simulink model "OBS6impedance"  (Simulink 7.4)
settings: Solver=ode45  StartTime=0.0  StopTime=8  MinStep=0.01  RelTol=1e-3
values from neighbouring files (symbols this model uses):
  Kact = eye(7)    [batchwamobs.m]
  Kd = Kp.^0.5*2    [WAMforcecontrol.m]    (also in batchwamobs.m = 50*eye(7); paralelcontrol2R.m = eye(n)*1000)
  Kp = 25*eye(7)    [batchwamobs.m]    (also in paralelcontrol2R.m = eye(n)*2500)
undefined symbols (not defined in the file or in its folder): Kf, Kif, Mdi, model1, model2, model3, model4, model5, model6, ncalculest, p560, uextgeneratorwall
libraries: roblocks x2
settings Model: Creator=acolome  LastModifiedBy=acolome

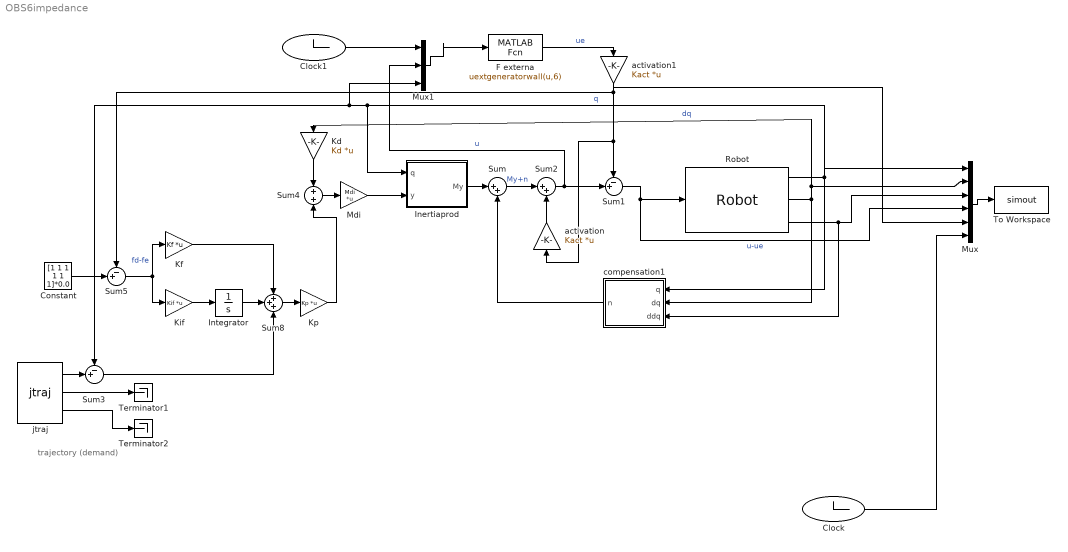
== system OBS6impedance ==
  note: trajectory
      | (demand)
  Clock : Clock
      settings: Decimation=100
  Clock1 : Clock
      settings: Decimation=100
  Constant : Constant  Value=[1 1 1 1 1 1]*0.0  OutDataType=fixdt(1, 16)  OutScaling=2^0
  F externa : MATLABFcn  MATLABFcn=uextgeneratorwall(u,6)  OutputDimensions=6
  Inertiaprod : Subsystem  mask{robot=p560, g=[0 0 9.81]}
      mask prompts: robot "Robot Object"; g "Gravity"
      mask init:
      | n=robot.n
      mask Display:
      | port_label('output',1,'M(q)y')
      | 
      | port_label('input', 1, 'q')
      | port_label('input', 2, 'y')
  Integrator : Integrator
  Kd : Gain  Gain=Kd  Multiplication=Matrix(K*u)  SaturateOnIntegerOverflow=on  OutDataTypeStr=Inherit: Same as input  ParamDataTypeStr=Inherit: Same as input
  Kf : Gain  Gain=Kf  Multiplication=Matrix(K*u)  SaturateOnIntegerOverflow=on  OutDataTypeStr=Inherit: Same as input  ParamDataTypeStr=Inherit: Same as input
  Kif : Gain  Gain=Kif  Multiplication=Matrix(K*u)  SaturateOnIntegerOverflow=on  OutDataTypeStr=Inherit: Same as input  ParamDataTypeStr=Inherit: Same as input
  Kp : Gain  Gain=Kp  Multiplication=Matrix(K*u)  SaturateOnIntegerOverflow=on  OutDataTypeStr=Inherit: Same as input  ParamDataTypeStr=Inherit: Same as input
  Mdi : Gain  Gain=Mdi  Multiplication=Matrix(K*u)  SaturateOnIntegerOverflow=on  OutDataTypeStr=Inherit: Same as input  ParamDataTypeStr=Inherit: Same as input
  Mux : Mux  Inputs=6
  Mux1 : Mux  Inputs=3
  Robot : roblocks/Robot  SystemSampleTime=-1  robot=p560  q0=[0 0 0 0 0 pi/20]*0
  Sum : Sum  Inputs=|++  OutDataType=fixdt(1, 16)  OutScaling=2^0
  Sum1 : Sum  Inputs=-+|  OutDataType=fixdt(1, 16)  OutScaling=2^0
  Sum2 : Sum  Inputs=|++  OutDataType=fixdt(1, 16)  OutScaling=2^0
  Sum3 : Sum  Inputs=-+|  SaturateOnIntegerOverflow=on  InputSameDT=on  OutDataTypeStr=Inherit: Same as first input
  Sum4 : Sum  SaturateOnIntegerOverflow=on  InputSameDT=on  OutDataTypeStr=Inherit: Same as first input
  Sum5 : Sum  Inputs=-+|  SaturateOnIntegerOverflow=on  InputSameDT=on  OutDataTypeStr=Inherit: Same as first input
  Sum8 : Sum  Inputs=+++  SaturateOnIntegerOverflow=on  InputSameDT=on  OutDataTypeStr=Inherit: Same as first input
  Terminator1 : Terminator
  Terminator2 : Terminator
  To Workspace : ToWorkspace  VariableName=simout  SampleTime=-1  SaveFormat=Array
  activation : Gain  Gain=Kact  Multiplication=Matrix(K*u)  SaturateOnIntegerOverflow=on  OutDataTypeStr=Inherit: Same as input  ParamDataTypeStr=Inherit: Same as input
  activation1 : Gain  Gain=Kact  Multiplication=Matrix(K*u)  SaturateOnIntegerOverflow=on  OutDataTypeStr=Inherit: Same as input  ParamDataTypeStr=Inherit: Same as input
  compensation1 : Subsystem  mask{robot=p560, g=[0 0 9.81], model1=model1, model2=model2, model3=model3, model4=model4, model5=model5, model6=model6}
      mask prompts: robot "Robot Object"; g "Gravity"; model1 "n1"; model2 "n2"; model3 "n3"; model4 "n4"; model5 "n5"; model6 "n6"
      mask init:
      | n=robot.n
      mask Display:
      | port_label('output',1,'n(q,dq)')
      | 
      | port_label('input', 1, 'q')
      | port_label('input', 2, 'dq')
      | port_label('input', 3, 'ddq')
  jtraj : roblocks/jtraj  SystemSampleTime=-1  q0=[0 0 0 0 0 pi/20]*0  qf=[1 1 1 1 1 1]  tmax=3
      link override MATLAB Fcn: MATLABFcn=squeeze(interp1(t,q,u))
      link override MATLAB Fcn1: MATLABFcn=squeeze(interp1(t,qd,u))
      link override MATLAB Fcn2: MATLABFcn=squeeze(interp1(t,qdd,u))
  wires:
  Mux/1 -> To Workspace/1
  jtraj/1 -> Sum3/2
  Robot/1 -> Mux/1, compensation1/1(q), Inertiaprod/1(q), Sum3/1, Mux1/3  "q"
  Robot/2 -> compensation1/2(dq), Mux/2, Kd/1  "dq"
  Robot/3 -> Mux/3, compensation1/3(ddq)
  compensation1/1(n) -> Sum/2
  Sum1/1 -> Robot/1, Mux/4  "u-ue"
  Inertiaprod/1(My) -> Sum/1
  Sum/1 -> Sum2/1  "My+n"
  Sum2/1 -> Sum1/2, Mux1/2  "u"
  F externa/1 -> activation1/1  "ue"
  activation1/1 -> Sum5/1, Sum1/1, activation/1, Mux/5
  activation/1 -> Sum2/2
  Constant/1 -> Sum5/2
  Sum5/1 -> Kf/1, Kif/1  "fd-fe"
  Kif/1 -> Integrator/1
  Kf/1 -> Sum8/1
  Integrator/1 -> Sum8/2
  jtraj/2 -> Terminator1/1
  jtraj/3 -> Terminator2/1
  Sum3/1 -> Sum8/3
  Sum8/1 -> Kp/1
  Kp/1 -> Sum4/2
  Kd/1 -> Sum4/1
  Sum4/1 -> Mdi/1
  Mdi/1 -> Inertiaprod/2(y)
  Mux1/1 -> F externa/1
  Clock1/1 -> Mux1/1
  Clock/1 -> Mux/6

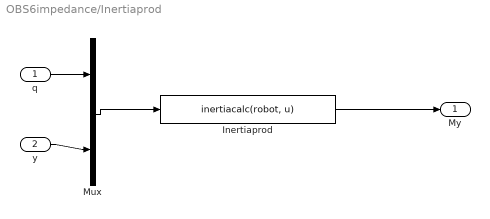
== system OBS6impedance/Inertiaprod ==
  q : Inport  OutDataType=fixdt(1, 16)  OutScaling=2^0
  y : Inport  Port=2  OutDataType=fixdt(1, 16)  OutScaling=2^0
  Inertiaprod : MATLABFcn  MATLABFcn=inertiacalc(robot, u)  OutputDimensions=n
  Mux : Mux  Inputs=2
  My : Outport  OutDataType=fixdt(1, 16)  OutScaling=2^0
  wires:
  Mux/1 -> Inertiaprod/1
  q/1 -> Mux/1
  Inertiaprod/1 -> My/1
  y/1 -> Mux/2

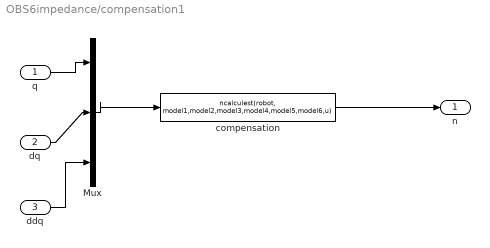
== system OBS6impedance/compensation1 ==
  q : Inport  OutDataType=fixdt(1, 16)  OutScaling=2^0
  dq : Inport  Port=2  OutDataType=fixdt(1, 16)  OutScaling=2^0
  ddq : Inport  Port=3  OutDataType=fixdt(1, 16)  OutScaling=2^0
  Mux : Mux  Inputs=3
  compensation : MATLABFcn  MATLABFcn=ncalculest(robot, model1,model2,model3,model4,model5,model6,u)  OutputDimensions=n
  n : Outport  OutDataType=fixdt(1, 16)  OutScaling=2^0
  wires:
  Mux/1 -> compensation/1
  q/1 -> Mux/1
  compensation/1 -> n/1
  dq/1 -> Mux/2
  ddq/1 -> Mux/3
